simulink model "MI_controle_W_I"  (R2015a)
settings: Solver=ode45  StartTime=0.0  StopTime=1.0  RelTol=1e-3
values from neighbouring files (symbols this model uses):
  FLrd_0 = FLr_dq_0    [MI_controle_W_I_T_inicio.m]    (also in MI_controle_W_I_inicio.m; MI_controle_W_I_startup_inicio.m; MI_controle_W_Inicio.m; MI_controle_W_T_I_startup_inicio.m)
  FLsd_0 = FluxLinkage_dq(1)    [MI_controle_W_I_T_inicio.m]    (also in MI_controle_W_I_inicio.m; MI_controle_W_I_startup_inicio.m; MI_controle_W_Inicio.m; MI_controle_W_T_I_startup_inicio.m)
  FLsq_0 = FluxLinkage_dq(2)    [MI_controle_W_I_T_inicio.m]    (also in MI_controle_W_I_inicio.m; MI_controle_W_I_startup_inicio.m; MI_controle_W_Inicio.m; MI_controle_W_T_I_startup_inicio.m)
  Isd_0 = Idq_0(1)    [MI_controle_W_I_T_inicio.m]    (also in MI_controle_W_I_inicio.m; MI_controle_W_I_startup_inicio.m; MI_controle_W_Inicio.m; MI_controle_W_T_I_startup_inicio.m)
  Isq_0 = Idq_0(2)    [MI_controle_W_I_T_inicio.m]    (also in MI_controle_W_I_inicio.m; MI_controle_W_I_startup_inicio.m; MI_controle_W_Inicio.m; MI_controle_W_T_I_startup_inicio.m)
  J = 0.025    [MI_controle_W_I_T_inicio.m]    (also in MI_controle_W_I_inicio.m; MI_controle_W_I_startup_inicio.m; MI_controle_W_Inicio.m; MI_controle_W_T_I_startup_inicio.m)
  Ki = (Wc^2*J)/(k*sqrt(1+tan(MF)^2))    [MI_controle_W_I_T_inicio.m]    (also in MI_controle_W_I_inicio.m; MI_controle_W_I_startup_inicio.m; MI_controle_W_Inicio.m; MI_controle_W_T_I_startup_inicio.m)
  Kii = Wci*(Wci*sigma*Ls + Rs*tanMF)/sqrt(tanMF^2 + 1)    [MI_controle_W_I_T_inicio.m]    (also in MI_controle_W_I_inicio.m; MI_controle_W_I_startup_inicio.m; MI_controle_W_T_I_startup_inicio.m = Wci*(Wci*sigma*Ls + Rs*tanMFi)/sqrt(tanMFi^2 + 1))
  Kp = Ki*tan(MF)/Wc    [MI_controle_W_I_T_inicio.m]    (also in MI_controle_W_I_inicio.m; MI_controle_W_I_startup_inicio.m; MI_controle_W_Inicio.m; MI_controle_W_T_I_startup_inicio.m)
  Kpi = (Kii/Wci)*(Wci*sigma*Ls*tanMF - Rs)/(Wci*sigma*Ls + Rs*tanMF)    [MI_controle_W_I_T_inicio.m]    (also in MI_controle_W_I_inicio.m; MI_controle_W_I_startup_inicio.m; MI_controle_W_T_I_startup_inicio.m = (Kii/Wci)*(Wci*sigma*Ls*tanMFi - Rs)/(Wci*sigma*Ls + Rs*tanM)
  Lm = Xm/Wsyn    (= 0.368708951496)    [MI_controle_W_I_T_inicio.m]    (also in MI_controle_W_I_inicio.m; MI_controle_W_I_startup_inicio.m; MI_controle_W_Inicio.m; MI_controle_W_T_I_startup_inicio.m)
  Lr = (Xlr + Xm)/Wsyn    (= 0.380831252995)    [MI_controle_W_I_T_inicio.m]    (also in MI_controle_W_I_inicio.m; MI_controle_W_I_startup_inicio.m; MI_controle_W_Inicio.m; MI_controle_W_T_I_startup_inicio.m)
  Minv = inv(M)    [MI_controle_W_I_T_inicio.m]    (also in MI_controle_W_I_inicio.m; MI_controle_W_I_startup_inicio.m; MI_controle_W_Inicio.m; MI_controle_W_T_I_startup_inicio.m)
  p = 4    [MI_controle_W_I_T_inicio.m]    (also in MI_controle_W_I_inicio.m; MI_controle_W_I_startup_inicio.m; MI_controle_W_Inicio.m; MI_controle_W_T_I_startup_inicio.m)
  Rs = 1.77    [MI_controle_W_I_T_inicio.m]    (also in MI_controle_W_I_inicio.m; MI_controle_W_I_startup_inicio.m; MI_controle_W_Inicio.m; MI_controle_W_T_I_startup_inicio.m)
  tau_r = Lr/Rr    (= 0.284202427608)    [MI_controle_W_I_T_inicio.m]    (also in MI_controle_W_I_inicio.m; MI_controle_W_I_startup_inicio.m; MI_controle_W_Inicio.m; MI_controle_W_T_I_startup_inicio.m)
  TL_0 = Tem_0    [MI_controle_W_I_T_inicio.m]    (also in MI_controle_W_I_inicio.m; MI_controle_W_I_startup_inicio.m = 0; MI_controle_W_Inicio.m; MI_controle_W_T_I_startup_inicio.m = 0)
  Wmech_0 = (2/p)*(1-s)*Wsyn    (= 185.253435597)    [MI_controle_W_I_T_inicio.m]    (also in MI_controle_W_I_inicio.m; MI_controle_W_I_startup_inicio.m = 0; MI_controle_W_Inicio.m; MI_controle_W_T_I_startup_inicio.m = 0)
undefined symbols (not defined in the file or in its folder): thetar
settings Model: Creator=range  LastModifiedBy=range

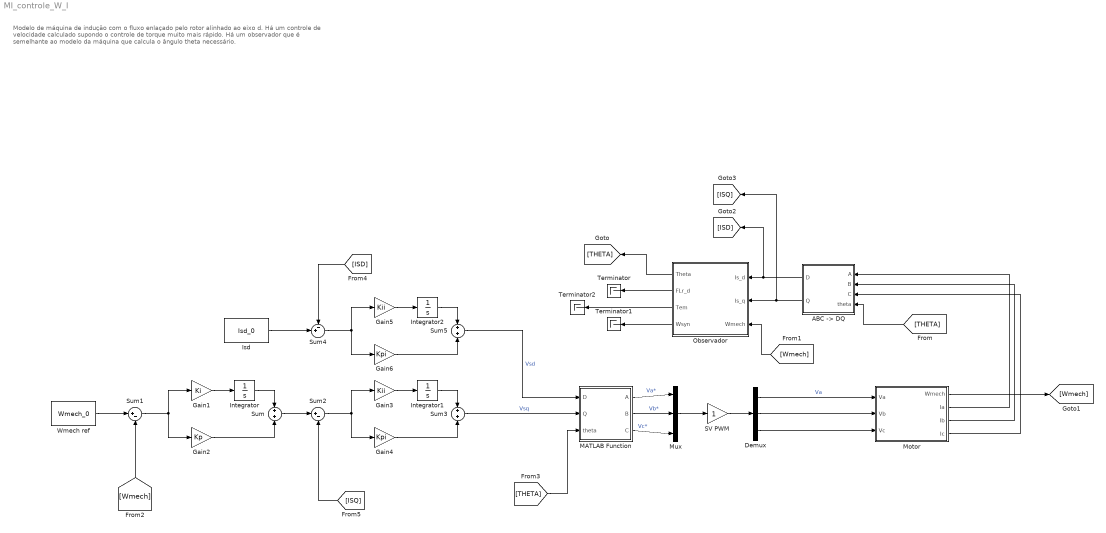
== system MI_controle_W_I ==
  note: Modelo de máquina de indução
      | com o fluxo enlaçado pelo rotor alinhado
      | ao eixo d.
      | Há um controle de velocidade calculado supondo o
      | controle de torque muito mais rápido.
      | Há um observador que é semelhante ao modelo da máquina
      | que calcula o ângulo theta necessário.
  "ABC -> DQ" : MATLAB Function  TreatAsAtomicUnit=on
  Demux : Demux  Outputs=3
  Gain1 : Gain  Gain=Ki
  Gain2 : Gain  Gain=Kp
  Gain3 : Gain  Gain=Kii
  Gain4 : Gain  Gain=Kpi
  Gain5 : Gain  Gain=Kii
  Gain6 : Gain  Gain=Kpi
  Integrator : Integrator  InitialCondition=Isq_0
  Integrator1 : Integrator  InitialCondition=Isq_0
  Integrator2 : Integrator  InitialCondition=Isq_0
  Isd : Constant  Value=Isd_0
  MATLAB Function : MATLAB Function  TreatAsAtomicUnit=on
  Motor : Subsystem
  Mux : Mux  Inputs=3
  Observador : Subsystem
  SV PWM : Gain
  Sum : Sum  Inputs=+|+
  Sum1 : Sum  Inputs=|+-
  Sum2 : Sum  Inputs=|+-
  Sum3 : Sum  Inputs=+|+
  Sum4 : Sum  Inputs=-+|
  Sum5 : Sum  Inputs=+|+
  Terminator : Terminator
  Terminator1 : Terminator
  Terminator2 : Terminator
  Wmech ref : Constant  Value=Wmech_0
  wires:
  "ABC -> DQ"/1(D) -> [ISD], Observador/1(Is_d)
  "ABC -> DQ"/2(Q) -> [ISQ], Observador/2(Is_q)
  Observador/2(FLr_d) -> Terminator/1
  Observador/4(Wsyn) -> Terminator1/1
  MATLAB Function/1(A) -> Mux/1  "Va*"
  MATLAB Function/2(B) -> Mux/2  "Vb*"
  MATLAB Function/3(C) -> Mux/3  "Vc*"
  Demux/1 -> Motor/1(Va)  "Va"
  Demux/2 -> Motor/2(Vb)
  Demux/3 -> Motor/3(Vc)
  Mux/1 -> SV PWM/1
  SV PWM/1 -> Demux/1
  Gain1/1 -> Integrator/1
  Integrator/1 -> Sum/1
  Gain2/1 -> Sum/2
  Wmech ref/1 -> Sum1/1
  Sum1/1 -> Gain1/1, Gain2/1
  Observador/1(Theta) -> [THETA]
  [THETA] -> "ABC -> DQ"/4(theta)
  Motor/1(Wmech) -> [Wmech]
  [Wmech] -> Observador/3(Wmech)
  [Wmech] -> Sum1/2
  [THETA] -> MATLAB Function/3(theta)
  Observador/3(Tem) -> Terminator2/1
  Sum/1 -> Sum2/1
  Gain3/1 -> Integrator1/1
  Integrator1/1 -> Sum3/1
  Gain4/1 -> Sum3/2
  Sum2/1 -> Gain3/1, Gain4/1
  Sum3/1 -> MATLAB Function/2(Q)  "Vsq"
  Gain5/1 -> Integrator2/1
  Integrator2/1 -> Sum5/1
  Gain6/1 -> Sum5/2
  Sum4/1 -> Gain5/1, Gain6/1
  Sum5/1 -> MATLAB Function/1(D)  "Vsd"
  Isd/1 -> Sum4/2
  [ISD] -> Sum4/1
  [ISQ] -> Sum2/2
  Motor/2(Ia) -> "ABC -> DQ"/1(A)
  Motor/3(Ib) -> "ABC -> DQ"/2(B)
  Motor/4(Ic) -> "ABC -> DQ"/3(C)

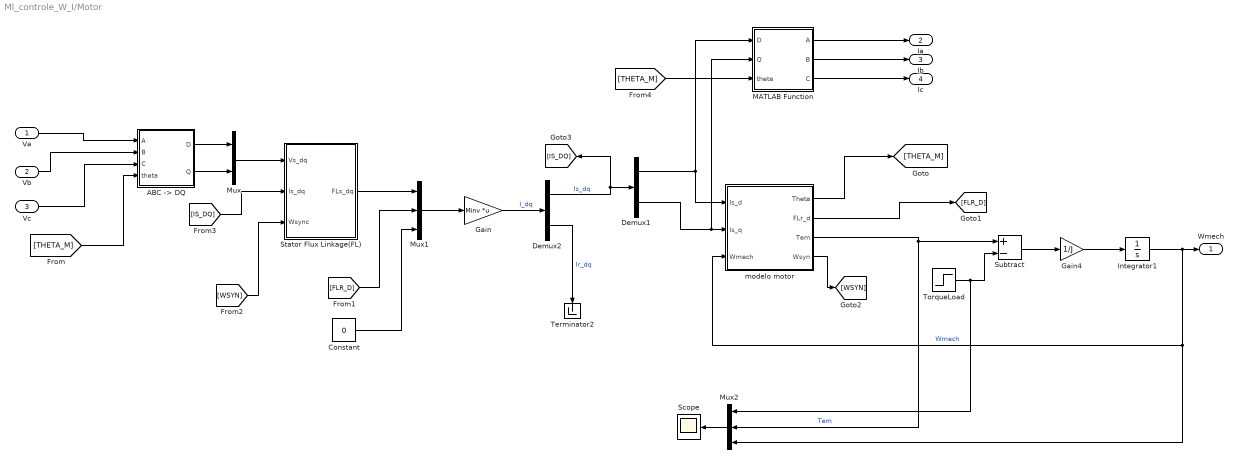
== system MI_controle_W_I/Motor ==
  Va : Inport
  Vb : Inport  Port=2
  Vc : Inport  Port=3
  "ABC -> DQ" : MATLAB Function  TreatAsAtomicUnit=on
  Constant : Constant  Value=0
  Demux1 : Demux  Outputs=2
  Demux2 : Demux  Outputs=2
  Gain : Gain  Gain=Minv  Multiplication=Matrix(K*u)
  Gain4 : Gain  Gain=1/J
  Integrator1 : Integrator  InitialCondition=Wmech_0
  MATLAB Function : MATLAB Function  TreatAsAtomicUnit=on
  Mux : Mux  Inputs=2
  Mux1 : Mux  Inputs=3
  Mux2 : Mux  Inputs=3
  Scope : Scope
  "Stator Flux Linkage(FL) " : Subsystem
  Subtract : Sum  Inputs=+-
  Terminator2 : Terminator
  TorqueLoad : Step  Time=0.5  Before=TL_0  After=TL_0/2  SampleTime=0
  modelo motor : Subsystem
  Wmech : Outport
  Ia : Outport  Port=2
  Ib : Outport  Port=3
  Ic : Outport  Port=4
  wires:
  Va/1 -> "ABC -> DQ"/1(A)
  Vb/1 -> "ABC -> DQ"/2(B)
  Vc/1 -> "ABC -> DQ"/3(C)
  modelo motor/2(FLr_d) -> [FLR_D]
  Mux2/1 -> Scope/1
  modelo motor/3(Tem) -> Mux2/2, Subtract/1  "Tem"
  Subtract/1 -> Gain4/1
  Gain4/1 -> Integrator1/1
  TorqueLoad/1 -> Subtract/2, Mux2/1
  Integrator1/1 -> modelo motor/3(Wmech), Mux2/3, Wmech/1  "Wmech"
  modelo motor/1(Theta) -> [THETA_M]
  [THETA_M] -> "ABC -> DQ"/4(theta)
  "ABC -> DQ"/1(D) -> Mux/1
  "ABC -> DQ"/2(Q) -> Mux/2
  Mux/1 -> "Stator Flux Linkage(FL) "/1(Vs_dq)
  Gain/1 -> Demux2/1  "I_dq"
  "Stator Flux Linkage(FL) "/1(FLs_dq) -> Mux1/1
  Demux2/2 -> Terminator2/1  "Ir_dq"
  Mux1/1 -> Gain/1
  [FLR_D] -> Mux1/2
  modelo motor/4(Wsyn) -> [WSYN]
  [WSYN] -> "Stator Flux Linkage(FL) "/3(Wsync)
  Constant/1 -> Mux1/3
  Demux2/1 -> [IS_DQ], Demux1/1  "Is_dq"
  Demux1/1 -> MATLAB Function/1(D), modelo motor/1(Is_d)
  Demux1/2 -> MATLAB Function/2(Q), modelo motor/2(Is_q)
  [IS_DQ] -> "Stator Flux Linkage(FL) "/2(Is_dq)
  [THETA_M] -> MATLAB Function/3(theta)
  MATLAB Function/1(A) -> Ia/1
  MATLAB Function/3(C) -> Ic/1
  MATLAB Function/2(B) -> Ib/1

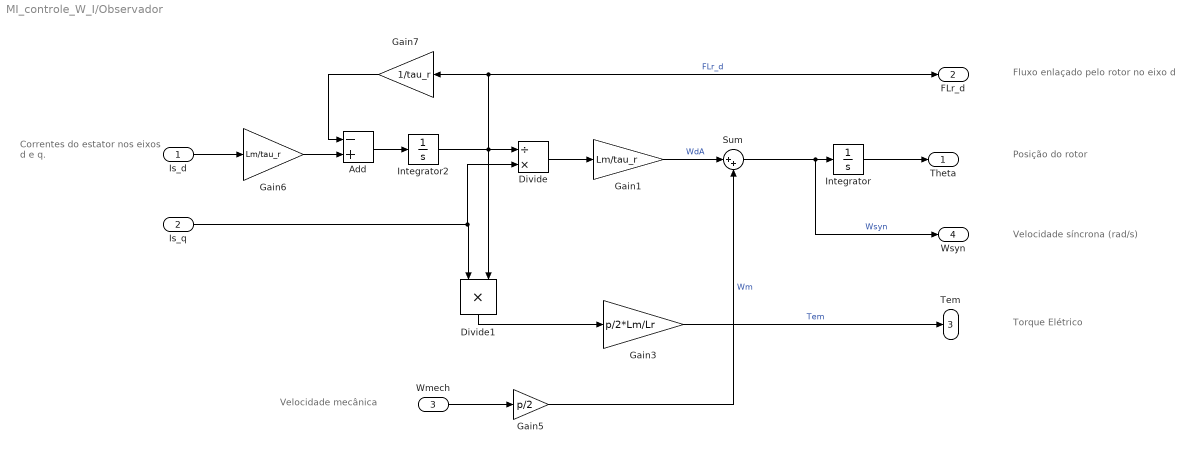
== system MI_controle_W_I/Observador ==
  note: Correntes do estator
      | nos eixos d e q.
  note: Velocidade mecânica
  note: Torque Elétrico
  note: Velocidade síncrona (rad/s)
  note: Posição do rotor
  note: Fluxo enlaçado pelo rotor no eixo d
  Is_d : Inport
  Is_q : Inport  Port=2
  Wmech : Inport  Port=3
  Add : Sum  Inputs=-+
  Divide : Product  Inputs=/*
  Divide1 : Product  Inputs=**
  Gain1 : Gain  Gain=Lm/tau_r
  Gain3 : Gain  Gain=p/2*Lm/Lr
  Gain5 : Gain  Gain=p/2
  Gain6 : Gain  Gain=Lm/tau_r
  Gain7 : Gain  Gain=1/tau_r
  Integrator : Integrator  InitialCondition=thetar
  Integrator2 : Integrator  InitialCondition=FLrd_0
  Sum : Sum  Inputs=|++
  Theta : Outport
  FLr_d : Outport  Port=2
  Tem : Outport  Port=3
  Wsyn : Outport  Port=4
  wires:
  Is_q/1 -> Divide/2, Divide1/1
  Integrator/1 -> Theta/1
  Sum/1 -> Wsyn/1, Integrator/1  "Wsyn"
  Add/1 -> Integrator2/1
  Gain1/1 -> Sum/1  "WdA"
  Is_d/1 -> Gain6/1
  Gain7/1 -> Add/1
  Gain6/1 -> Add/2
  Integrator2/1 -> Gain7/1, FLr_d/1, Divide1/2, Divide/1  "FLr_d"
  Divide1/1 -> Gain3/1
  Gain3/1 -> Tem/1  "Tem"
  Divide/1 -> Gain1/1
  Wmech/1 -> Gain5/1
  Gain5/1 -> Sum/2  "Wm"

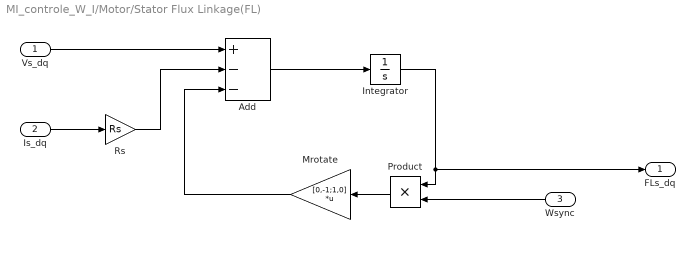
== system MI_controle_W_I/Motor/Stator Flux Linkage(FL)  ==
  Vs_dq : Inport
  Is_dq : Inport  Port=2
  Wsync : Inport  Port=3
  Add : Sum  Inputs=+--
  Integrator : Integrator  InitialCondition=[FLsd_0;FLsq_0]
  Mrotate : Gain  Gain=[0,-1;1,0]  Multiplication=Matrix(K*u)
  Product : Product
  Rs : Gain  Gain=Rs
  FLs_dq : Outport
  wires:
  Vs_dq/1 -> Add/1
  Product/1 -> Mrotate/1
  Rs/1 -> Add/2
  Add/1 -> Integrator/1
  Mrotate/1 -> Add/3
  Integrator/1 -> FLs_dq/1, Product/1
  Wsync/1 -> Product/2
  Is_dq/1 -> Rs/1

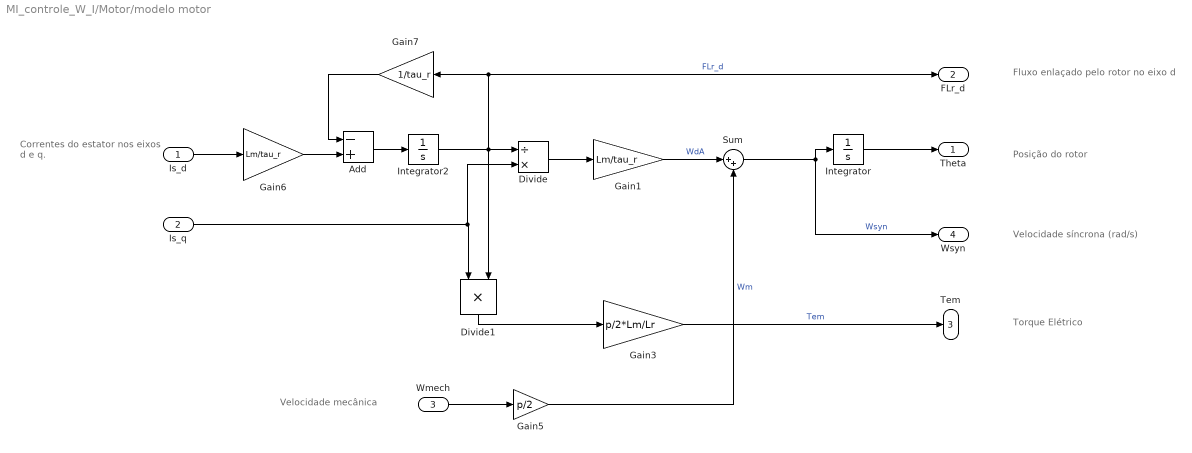
== system MI_controle_W_I/Motor/modelo motor ==
  note: Correntes do estator
      | nos eixos d e q.
  note: Velocidade mecânica
  note: Torque Elétrico
  note: Velocidade síncrona (rad/s)
  note: Posição do rotor
  note: Fluxo enlaçado pelo rotor no eixo d
  Is_d : Inport
  Is_q : Inport  Port=2
  Wmech : Inport  Port=3
  Add : Sum  Inputs=-+
  Divide : Product  Inputs=/*
  Divide1 : Product  Inputs=**
  Gain1 : Gain  Gain=Lm/tau_r
  Gain3 : Gain  Gain=p/2*Lm/Lr
  Gain5 : Gain  Gain=p/2
  Gain6 : Gain  Gain=Lm/tau_r
  Gain7 : Gain  Gain=1/tau_r
  Integrator : Integrator  InitialCondition=thetar
  Integrator2 : Integrator  InitialCondition=FLrd_0
  Sum : Sum  Inputs=|++
  Theta : Outport
  FLr_d : Outport  Port=2
  Tem : Outport  Port=3
  Wsyn : Outport  Port=4
  wires:
  Is_q/1 -> Divide/2, Divide1/1
  Integrator/1 -> Theta/1
  Sum/1 -> Wsyn/1, Integrator/1  "Wsyn"
  Add/1 -> Integrator2/1
  Gain1/1 -> Sum/1  "WdA"
  Is_d/1 -> Gain6/1
  Gain7/1 -> Add/1
  Gain6/1 -> Add/2
  Integrator2/1 -> Gain7/1, FLr_d/1, Divide1/2, Divide/1  "FLr_d"
  Divide1/1 -> Gain3/1
  Gain3/1 -> Tem/1  "Tem"
  Divide/1 -> Gain1/1
  Wmech/1 -> Gain5/1
  Gain5/1 -> Sum/2  "Wm"

== matlab function MI_controle_W_I/ABC -> DQ ==
  data: A input; D output; B input; C input; theta input; Q output
function [D,Q] = ABCtoDQ(A,B,C,theta)
%Transformação de grandezas trifásicas para os eixos D e Q.

DQ = sqrt(2/3)*[cos(theta), cos(theta-2*pi/3), cos(theta-4*pi/3);...
               -sin(theta),-sin(theta-2*pi/3),-sin(theta-4*pi/3)]*[A;B;C];
D = DQ(1);
Q = DQ(2);

== matlab function MI_controle_W_I/Motor/ABC -> DQ ==
  data: A input; D output; B input; C input; theta input; Q output
function [D,Q] = ABCtoDQ(A,B,C,theta)
%Transformação de grandezas trifásicas para os eixos D e Q.

DQ = sqrt(2/3)*[cos(theta), cos(theta-2*pi/3), cos(theta-4*pi/3);...
               -sin(theta),-sin(theta-2*pi/3),-sin(theta-4*pi/3)]*[A;B;C];
D = DQ(1);
Q = DQ(2);

== matlab function MI_controle_W_I/MATLAB Function ==
  data: D input; A output; Q input; theta input; B output; C output
function [A,B,C] = DQtoABC(D,Q,theta)
%Transformação inversa de Park.

ABC = sqrt(2/3)*[cos(theta),          -sin(theta); ...
                 cos(theta + 4*pi/3), -sin(theta + 4*pi/3); ...
                 cos(theta + 2*pi/3), -sin(theta + 2*pi/3)]*[D;Q];
A = ABC(1);
B = ABC(2);
C = ABC(3);

== matlab function MI_controle_W_I/Motor/MATLAB Function ==
  data: D input; A output; Q input; theta input; B output; C output
function [A,B,C] = DQtoABC(D,Q,theta)
%Transformação inversa de Park.

ABC = sqrt(2/3)*[cos(theta),          -sin(theta); ...
                 cos(theta + 4*pi/3), -sin(theta + 4*pi/3); ...
                 cos(theta + 2*pi/3), -sin(theta + 2*pi/3)]*[D;Q];
A = ABC(1);
B = ABC(2);
C = ABC(3);
